simulink model "xEMU_SimulationModel3_rule1"  (R2017b)
settings: Solver=ode4  StartTime=0.0  StopTime=8192  FixedStep=0.01  RelTol=1e-3
undefined symbols (not defined in the file): a1, a2, a3, a4, ACO, BAT, Battery, DCT, DRT, EMS, ENV, Fahrzyklus_VS_modell, height_BAT, leistung, lib_bat, Maximum, Maximum_position, Num_cells, P_FC_max_long, P_FC_min_long, P_FC_step_max, Pbat_charge_max, Pbat_discharge_max, Pfc_max, Pfc_min, SOC_tar, time_peaks, TRM, velocity_peaks
libraries: simulink x5
(part 3 of 15)

== system xEMU_SimulationModel3_rule1/Battery (BAT)_mittel_02/Cell/Thermal ==
  CellToFV : Subsystem
  ConductivityMatrix : MATLAB Function  TreatAsAtomicUnit=on
  Coolings : Subsystem
  FV Temperatures : Integrator  ExternalReset=rising  InitialCondition=[ MDL.battery.initialState.CellElement_1.temperature MDL.battery.initialState.CellElement_1.temperature MDL.battery.initialState.CellElement_1.temperature MDL.battery.initialState.CellElement_1.temperature MDL.battery.initialState.CellElement_1.temperature MDL.battery.initialState.CellElement_1.temperature MDL.battery.initialState.CellElement_1.temperature MDL.battery.initialState.CellElement_1.temperature MDL.battery.initialState.CellElement_1.temperature MDL.battery.initialState.CellElement_1.temperature MDL.battery.initialState.CellElement_1.temperature MDL.battery.initialState.CellElement_1.temperature MDL.battery.initialState.CellElement_1.temperature MDL.battery.initialState.CellElement_1.temperature MDL.battery.initialState.CellElement_1.temperature MDL.battery.initialState.CellElement_1.temperature MDL.battery.initialState.CellElement_1.temperature MDL.battery.initialState.CellElement_1.temperature MDL.battery.initialState.CellElement_1.temperature MDL.battery.initialState.CellElement_1.temperature MDL.battery.initialState.CellElement_1.temperature MDL.battery.initialState.CellElement_1.temperature MDL.battery.initialState.CellElement_1.temperature MDL.battery.initialState.CellElement_1.temperature MDL.battery.initialState.CellElement_1.temperature MDL.battery.initialState.CellElement_1.temperature MDL.battery.initialState.CellElement_1.temperature MDL.battery.initialState.CellElement_1.temperature MDL.battery.initialState.CellElement_1.temperature MDL.battery.initialState.CellElement_1.temperature MDL.battery.initialState.CellElement_1.temperature MDL.battery.initialState.CellElement_1.temperature MDL.battery.initialState.CellElement_1.temperature MDL.battery.initialState.CellElement_1.temperature MDL.battery.initialState.CellElement_1.temperature MDL.battery.initialState.CellElement_1.temperature MDL.battery.initialState.CellElement_1.temperature MDL.battery.initialState.CellElement_1.temperature MDL.battery.initialState.CellElement_1.temperature MDL.battery.initialState.CellElement_1.temperature MDL.battery.initialState.CellElement_1.temperature MDL.battery.initialState.CellElement_1.temperature MDL.battery.initialState.CellElement_1.temperature MDL.battery.initialState.CellElement_1.temperature MDL.battery.initialState.CellElement_1.temperature MDL.battery.initialState.CellElement_1.temperature MDL.battery.initialState.CellElement_1.temperature MDL.battery.initialState.CellElement_1.temperature MDL.battery.initialState.CellElement_1.temperature MDL.battery.initialState.CellElement_1.temperature MDL.battery.initialState.CellElement_1.temperature MDL.battery.initialState.CellElement_1.temperature MDL.battery.initialState.CellElement_1.temperature MDL.battery.initialState.CellElement_1.temperature MDL.battery.initialState.CellElement_1.temperature MDL.battery.initialState.CellElement_1.temperature MDL.battery.initialState.CellElement_1.temperature MDL.battery.initialState.CellElement_1.temperature MDL.battery.initialState.CellElement_1.temperature MDL.battery.initialState.CellElement_1.temperature MDL.battery.initialState.CellElement_1.temperature MDL.battery.initialState.CellElement_1.temperature MDL.battery.initialState.CellElement_1.temperature MDL.battery.initialState.CellElement_1.temperature MDL.battery.initialState.CellElement_1.temperature MDL.battery.initialState.CellElement_1.temperature MDL.battery.initialState.CellElement_1.temperature MDL.battery.initialState.CellElement_1.temperature MDL.battery.initialState.CellElement_1.temperature MDL.battery.initialState.CellElement_1.temperature MDL.battery.initialState.CellElement_1.temperature MDL.battery.initialState.CellElement_1.temperature MDL.battery.initialState.CellElement_1.temperature MDL.battery.initialState.CellElement_1.temperature MDL.battery.initialState.CellElement_1.temperature MDL.battery.initialState.CellElement_1.temperature MDL.battery.initialState.CellElement_1.temperature MDL.battery.initialState.CellElement_1.temperature MDL.battery.initialState.CellElement_1.temperature MDL.battery.initialState.CellElement_1.temperature MDL.battery.initialState.CellElement_1.temperature MDL.battery.initialState.CellElement_1.temperature MDL.battery.initialState.CellElement_1.temperature MDL.battery.initialState.CellElement_1.temperature MDL.battery.initialState.CellElement_1.temperature MDL.battery.initialState.CellElement_1.temperature MDL.battery.initialState.CellElement_1.temperature MDL.battery.initialState.CellElement_1.temperature MDL.battery.initialState.CellElement_1.temperature MDL.battery.initialState.CellElement_1.temperature MDL.battery.initialState.CellElement_1.temperature MDL.battery.initialState.CellElement_1.temperature MDL.battery.initialState.CellElement_1.temperature MDL.battery.initialState.CellElement_1.temperature MDL.battery.initialState.CellElement_1.temperature MDL.battery.initialState.CellElement_1.temperature MDL.battery.initialState.CellElement_1.temperature MDL.battery.initialState.CellElement_1.temperature MDL.battery.initialState.CellElement_1.temperature MDL.battery.initialState.CellElement_1.temperature MDL.battery.initialState.CellElement_1.temperature MDL.battery.initialState.CellElement_1.temperature MDL.battery.initialState.CellElement_1.temperature MDL.battery.initialState.CellElement_1.temperature MDL.battery.initialState.CellElement_1.temperature MDL.battery.initialState.CellElement_1.temperature MDL.battery.initialState.CellElement_1.temperature MDL.battery.initialState.CellElement_1.temperature MDL.battery.initialState.CellElement_1.temperature MDL.battery.initialState.CellElement_1.temperature MDL.battery.initialState.CellElement_1.temperature MDL.battery.initialState.CellElement_1.temperature MDL.battery.initialState.CellElement_1.temperature MDL.battery.initialState.CellElement_1.temperature MDL.battery.initialState.CellElement_1.temperature MDL.battery.initialState.CellElement_1.temperature MDL.battery.initialState.CellElement_1.temperature MDL.battery.initialState.CellElement_1.temperature MDL.battery.initialState.CellElement_1.temperature MDL.battery.initialState.CellElement_1.temperature MDL.battery.initialState.CellElement_1.temperature MDL.battery.initialState.CellElement_1.temperature MDL.battery.initialState.CellElement_1.temperature MDL.battery.initialState.CellElement_1.temperature MDL.battery.initialState.CellElement_1.temperature MDL.battery.initialState.CellElement_1.temperature MDL.battery.initialState.CellElement_1.temperature MDL.battery.initialState.CellElement_1.temperature MDL.battery.initialState.CellElement_1.temperature MDL.battery.initialState.CellElement_1.temperature MDL.battery.initialState.CellElement_1.temperature MDL.battery.initialState.CellElement_1.temperature MDL.battery.initialState.CellElement_1.temperature MDL.battery.initialState.CellElement_1.temperature MDL.battery.initialState.CellElement_1.temperature MDL.battery.initialState.CellElement_1.temperature MDL.battery.initialState.CellElement_1.temperature MDL.battery.initialState.CellElement_1.temperature MDL.battery.initialState.CellElement_1.temperature MDL.battery.initialState.CellElement_1.temperature MDL.battery.initialState.CellElement_1.temperature MDL.battery.initialState.CellElement_1.temperature MDL.battery.initialState.CellElement_1.temperature MDL.battery.initialState.CellElement_1.temperature MDL.battery.initialState.CellElement_1.temperature MDL.battery.initialState.CellElement_1.temperature MDL.battery.initialState.CellElement_1.temperature MDL.battery.initialState.CellElement_1.temperature MDL.battery.initialState.CellElement_1.temperature MDL.battery.initialState.CellElement_1.temperature MDL.battery.initialState.CellElement_1.temperature MDL.battery.initialState.CellElement_1.temperature MDL.battery.initialState.CellElement_1.temperature MDL.battery.initialState.CellElement_1.temperature MDL.battery.initialState.CellElement_1.temperature MDL.battery.initialState.CellElement_1.temperature MDL.battery.initialState.CellElement_1.temperature MDL.battery.initialState.CellElement_1.temperature MDL.battery.initialState.CellElement_1.temperature MDL.battery.initialState.CellElement_1.temperature MDL.battery.initialState.CellElement_1.temperature MDL.battery.initialState.CellElement_1.temperature MDL.battery.initialState.CellElement_1.temperature MDL.battery.initialState.CellElement_1.temperature MDL.battery.initialState.CellElement_1.temperature MDL.battery.initialState.CellElement_1.temperature MDL.battery.initialState.CellElement_1.temperature MDL.battery.initialState.CellElement_1.temperature MDL.battery.initialState.CellElement_1.temperature MDL.battery.initialState.CellElement_1.temperature MDL.battery.initialState.CellElement_1.temperature MDL.battery.initialState.CellElement_1.temperature MDL.battery.initialState.CellElement_1.temperature MDL.battery.initialState.CellElement_1.temperature MDL.battery.initialState.CellElement_1.temperature MDL.battery.initialState.CellElement_1.temperature MDL.battery.initialState.CellElement_1.temperature MDL.battery.initialState.CellElement_1.temperature MDL.battery.initialState.CellElement_1.temperature MDL.battery.initialState.CellElement_1.temperature MDL.battery.initialState.CellElement_1.temperature MDL.battery.initialState.CellElement_1.temperature MDL.battery.initialState.CellElement_1.temperature MDL.battery.initialState.CellElement_1.temperature MDL.battery.initialState.CellElement_1.temperature MDL.battery.initialState.CellElement_1.temperature MDL.battery.initialState.CellElement_1.temperature MDL.battery.initialState.CellElement_1.temperature MDL.battery.initialState.CellElement_1.temperature MDL.battery.initialState.CellElement_1.temperature MDL.battery.initialState.CellElement_1.temperature MDL.battery.initialState.CellElement_1.temperature MDL.battery.initialState.CellElement_1.temperature MDL.battery.initialState.CellElement_1.temperature MDL.battery.initialState.CellElement_1.temperature MDL.battery.initialState.CellElement_1.temperature MDL.battery.initialState.CellElement_1.temperature MDL.battery.initialState.CellElement_1.temperature MDL.battery.initialState.CellElement_1.temperature MDL.battery.initialState.CellElement_1.temperature MDL.battery.initialState.CellElement_1.temperature MDL.battery.initialState.CellElement_1.temperature MDL.battery.initialState.CellElement_1.temperature MDL.battery.initialState.CellElement_1.temperature MDL.battery.initialState.CellElement_1.temperature MDL.battery.initialState.CellElement_1.temperature MDL.battery.initialState.CellElement_1.temperature MDL.battery.initialState.CellElement_1.temperature MDL.battery.initialState.CellElement_1.temperature MDL.battery.initialState.CellElement_1.temperature MDL.battery.initialState.CellElement_1.temperature MDL.battery.initialState.CellElement_1.temperature MDL.battery.initialState.CellElement_1.temperature MDL.battery.initialState.CellElement_1.temperature MDL.battery.initialState.CellElement_1.temperature MDL.battery.initialState.CellElement_1.temperature MDL.battery.initialState.CellElement_1.temperature MDL.battery.initialState.CellElement_1.temperature MDL.battery.initialState.CellElement_1.temperature MDL.battery.initialState.CellElement_1.temperature MDL.battery.initialState.CellElement_1.temperature MDL.battery.initialState.CellElement_1.temperature MDL.battery.initialState.CellElement_1.temperature MDL.battery.initialState.CellElement_1.temperature MDL.battery.initialState.CellElement_1.temperature MDL.battery.initialState.CellElement_1.temperature MDL.battery.initialState.CellElement_1.temperature MDL.battery.initialState.CellElement_1.temperature MDL.battery.initialState.CellElement_1.temperature MDL.battery.initialState.CellElement_1.temperature MDL.battery.initialState.CellElement_1.temperature MDL.battery.initialState.CellElement_1.temperature MDL.battery.initialState.CellElement_1.temperature MDL.battery.initialState.CellElement_1.temperature MDL.battery.initialState.CellElement_1.temperature MDL.battery.initialState.CellElement_1.temperature MDL.battery.initialState.CellElement_1.temperature MDL.battery.initialState.CellElement_1.temperature MDL.battery.initialState.CellElement_1.temperature MDL.battery.initialState.CellElement_1.temperature MDL.battery.initialState.CellElement_1.temperature MDL.battery.initialState.CellElement_1.temperature MDL.battery.initialState.CellElement_1.temperature MDL.battery.initialState.CellElement_1.temperature MDL.battery.initialState.CellElement_1.temperature MDL.battery.initialState.CellElement_1.temperature MDL.battery.initialState.CellElement_1.temperature MDL.battery.initialState.CellElement_1.temperature MDL.battery.initialState.CellElement_1.temperature MDL.battery.initialState.CellElement_1.temperature MDL.battery.initialState.CellElement_1.temperature MDL.battery.initialState.CellElement_1.temperature MDL.battery.initialState.CellElement_1.temperature MDL.battery.initialState.CellElement_1.temperature MDL.battery.initialState.CellElement_1.temperature MDL.battery.initialState.CellElement_1.temperature MDL.battery.initialState.CellElement_1.temperature MDL.battery.initialState.CellElement_1.temperature MDL.battery.initialState.CellElement_1.temperature MDL.battery.initialState.CellElement_1.temperature MDL.battery.initialState.CellElement_1.temperature MDL.battery.initialState.CellElement_1.temperature MDL.battery.initialState.CellElement_1.temperature MDL.battery.initialState.CellElement_1.temperature MDL.battery.initialState.CellElement_1.temperature MDL.battery.initialState.CellElement_1.temperature MDL.battery.initialState.CellElement_1.temperature MDL.battery.initialState.CellElement_1.temperature MDL.battery.initialState.CellElement_1.temperature MDL.battery.initialState.CellElement_1.temperature MDL.battery.initialState.CellElement_1.temperature MDL.battery.initialState.CellElement_1.temperature MDL.battery.initialState.CellElement_1.temperature MDL.battery.initialState.CellElement_1.temperature MDL.battery.initialState.CellElement_1.temperature MDL.battery.initialState.CellElement_1.temperature MDL.battery.initialState.CellElement_1.temperature MDL.battery.initialState.CellElement_1.temperature MDL.battery.initialState.CellElement_1.temperature MDL.battery.initialState.CellElement_1.temperature MDL.battery.initialState.CellElement_1.temperature MDL.battery.initialState.CellElement_1.temperature MDL.battery.initialState.CellElement_1.temperature MDL.battery.initialState.CellElement_1.temperature MDL.battery.initialState.CellElement_1.temperature MDL.battery.initialState.CellElement_1.temperature MDL.battery.initialState.CellElement_1.temperature MDL.battery.initialState.CellElement_1.temperature MDL.battery.initialState.CellElement_1.temperature MDL.battery.initialState.CellElement_1.temperature MDL.battery.initialState.CellElement_1.temperature MDL.battery.initialState.CellElement_1.temperature MDL.battery.initialState.CellElement_1.temperature MDL.battery.initialState.CellElement_1.temperature MDL.battery.initialState.CellElement_1.temperature MDL.battery.initialState.CellElement_1.temperature MDL.battery.initialState.CellElement_1.temperature MDL.battery.initialState.CellElement_1.temperature MDL.battery.initialState.CellElement_1.temperature MDL.battery.initialState.CellElement_1.temperature ]
  FVToCell : Subsystem
  Reciprocals of Thermal Capacities : Gain  Gain=[0.582768314846317;0.582768314846317;0.582768314846317;0.582768314846317;0.582768314846317;0.582768314846317;0.582768314846317;0.582768314846317;0.582768314846317;0.582768314846317;0.582768314846317;0.582768314846317;0.582768314846317;0.582768314846317;0.582768314846317;0.582768314846317;0.582768314846317;0.582768314846317;0.582768314846317;0.582768314846317;0.582768314846317;0.582768314846317;0.582768314846317;0.582768314846317;0.582768314846317;0.582768314846317;0.582768314846317;0.582768314846317;0.582768314846317;0.582768314846317;0.582768314846317;0.582768314846317;0.582768314846317;0.582768314846317;0.582768314846317;0.582768314846317;0.582768314846317;0.582768314846317;0.582768314846317;0.582768314846317;0.582768314846317;0.582768314846317;0.582768314846317;0.582768314846317;0.582768314846317;0.582768314846317;0.582768314846317;0.582768314846317;0.582768314846317;0.582768314846317;0.582768314846317;0.582768314846317;0.582768314846317;0.582768314846317;0.582768314846317;0.582768314846317;0.582768314846317;0.582768314846317;0.582768314846317;0.582768314846317;0.582768314846317;0.582768314846317;0.582768314846317;0.582768314846317;0.582768314846317;0.582768314846317;0.582768314846317;0.582768314846317;0.582768314846317;0.582768314846317;0.582768314846317;0.582768314846317;0.582768314846317;0.582768314846317;0.582768314846317;0.582768314846317;0.582768314846317;0.582768314846317;0.582768314846317;0.582768314846317;0.582768314846317;0.582768314846317;0.582768314846317;0.582768314846317;0.582768314846317;0.582768314846317;0.582768314846317;0.582768314846317;0.582768314846317;0.582768314846317;0.582768314846317;0.582768314846317;0.582768314846317;0.582768314846317;0.582768314846317;0.582768314846317;0.582768314846317;0.582768314846317;0.582768314846317;0.582768314846317;0.582768314846317;0.582768314846317;0.582768314846317;0.582768314846317;0.582768314846317;0.582768314846317;0.582768314846317;0.582768314846317;0.582768314846317;0.582768314846317;0.582768314846317;0.582768314846317;0.582768314846317;0.582768314846317;0.582768314846317;0.582768314846317;0.582768314846317;0.582768314846317;0.582768314846317;0.582768314846317;0.582768314846317;0.582768314846317;0.582768314846317;0.582768314846317;0.582768314846317;0.582768314846317;0.582768314846317;0.582768314846317;0.582768314846317;0.582768314846317;0.582768314846317;0.582768314846317;0.582768314846317;0.582768314846317;0.582768314846317;0.582768314846317;0.582768314846317;0.582768314846317;0.582768314846317;0.582768314846317;0.582768314846317;0.582768314846317;0.582768314846317;0.582768314846317;0.582768314846317;0.582768314846317;0.582768314846317;0.582768314846317;0.582768314846317;0.582768314846317;0.582768314846317;0.582768314846317;0.582768314846317;0.582768314846317;0.582768314846317;0.582768314846317;0.582768314846317;0.582768314846317;0.582768314846317;0.582768314846317;0.582768314846317;0.582768314846317;0.582768314846317;0.582768314846317;0.582768314846317;0.582768314846317;0.582768314846317;0.582768314846317;0.582768314846317;0.582768314846317;0.582768314846317;0.582768314846317;0.582768314846317;0.582768314846317;0.582768314846317;0.582768314846317;0.582768314846317;0.582768314846317;0.582768314846317;0.582768314846317;0.582768314846317;0.582768314846317;0.582768314846317;0.582768314846317;0.582768314846317;0.582768314846317;0.582768314846317;0.582768314846317;0.582768314846317;0.582768314846317;0.582768314846317;0.582768314846317;0.582768314846317;0.582768314846317;0.582768314846317;0.582768314846317;0.582768314846317;0.582768314846317;0.582768314846317;0.582768314846317;0.582768314846317;0.582768314846317;0.582768314846317;0.582768314846317;0.582768314846317;0.582768314846317;0.582768314846317;0.582768314846317;0.582768314846317;0.582768314846317;0.582768314846317;0.582768314846317;0.582768314846317;0.582768314846317;0.582768314846317;0.582768314846317;0.582768314846317;0.582768314846317;0.582768314846317;0.582768314846317;0.582768314846317;0.582768314846317 ...(+1404 chars)]
  Sum : Sum  Inputs=|+-+
  wires:
  [Reset] -> FV Temperatures/2
  ConductivityMatrix/1(y) -> Sum/3
  CellToFV/1(P_FV) -> Sum/1
  Coolings/1(P_FV) -> Sum/2
  FV Temperatures/1 -> Coolings/1(T_FV), ConductivityMatrix/1(u), FVToCell/1(T_FV)
  Reciprocals of Thermal Capacities/1 -> FV Temperatures/1
  Sum/1 -> Reciprocals of Thermal Capacities/1

== system xEMU_SimulationModel3_rule1/Battery (BAT)_mittel_02/Cell/TotalValues ==
  Component0 : Subsystem
  Component1 : Subsystem
  Component2 : Subsystem
  Current : Outport
  Voltage : Outport  Port=2
  Power : Outport  Port=3
  wires:
  Component0/3(Value) -> Current/1
  Component1/3(Value) -> Voltage/1
  Component2/3(Value) -> Power/1

== system xEMU_SimulationModel3_rule1/DCDC Traction (DCT)/DCDC_elektrisch_Modellierung/Efficiency measurment ==
  In1 : Inport
  In2 : Inport  Port=2
  Abs : Abs
  Abs1 : Abs
  Clock : Clock
  Constant : Constant
  Constant1 : Constant  Value=0
  Divide : Product  Inputs=*/
  Divide1 : Product  Inputs=*/
  Divide2 : Product  Inputs=*/
  Integrator2 : Integrator
  Relational Operator : RelationalOperator  Operator=<=  OutDataTypeStr=boolean  RndMeth=Simplest
  Relational Operator1 : RelationalOperator  Operator===  OutDataTypeStr=boolean  RndMeth=Simplest
  Scope : Scope  NumInputPorts=4
  Switch : Switch  Criteria=u2 > Threshold
  Switch1 : Switch  Criteria=u2 > Threshold
  Efficiency : Outport
  wires:
  Abs/1 -> Divide/2, Divide1/1, Relational Operator/1
  In2/1 -> Scope/2, Abs1/1
  Abs1/1 -> Divide1/2, Relational Operator/2, Divide/1
  Switch1/1 -> Integrator2/1, Scope/4
  Relational Operator1/1 -> Switch1/2
  In1/1 -> Scope/1, Abs/1
  Divide1/1 -> Switch/1
  Divide/1 -> Switch/3
  Constant1/1 -> Relational Operator1/1
  Relational Operator/1 -> Switch/2
  Switch/1 -> Switch1/3, Relational Operator1/2, Scope/3
  Constant/1 -> Switch1/1
  Integrator2/1 -> Divide2/1
  Clock/1 -> Divide2/2
  Divide2/1 -> Efficiency/1

== system xEMU_SimulationModel3_rule1/DCDC Traction (DCT)/DCDC_elektrisch_Modellierung/Efficiency measurment1 ==
  In1 : Inport
  In2 : Inport  Port=2
  Abs : Abs
  Abs1 : Abs
  Divide3 : Product  Inputs=*/
  Integrator1 : Integrator
  Integrator3 : Integrator
  Sum : Sum  Inputs=|++
  Switch1 : Switch
  Switch2 : Switch
  Efficiency : Outport
  wires:
  In2/1 -> Sum/2
  Sum/1 -> Abs/1
  Abs1/1 -> Switch1/3, Switch2/1
  In1/1 -> Abs1/1, Switch2/2, Switch1/2, Sum/1
  Switch1/1 -> Integrator1/1
  Abs/1 -> Switch2/3, Switch1/1
  Switch2/1 -> Integrator3/1
  Integrator3/1 -> Divide3/1
  Integrator1/1 -> Divide3/2
  Divide3/1 -> Efficiency/1

== system xEMU_SimulationModel3_rule1/Drive Train (DRT)/Converter and traction motor/Converter_DRT ==
  "I_traction_motor " : Inport
  V_dcLinkStorage_V : Inport  Port=2
  V_Drive_V : Inport  Port=3
  Cos_Phi_Phaseshift : Inport  Port=4
  RPM : Inport  Port=5
  Clock : Clock
  Display : Display
  Divide2 : Product  Inputs=*/
  Gain : Gain  Gain=1/1000
  Gain3 : Gain  Gain=1/sqrt(3)
  Integrator2 : Integrator
  Sum : Sum  Inputs=|++
  n-D Lookup Diode : Lookup_n-D  NumberOfTableDimensions=4  BreakpointsForDimension1=DRT.converter.loss_diode.D1_U_Load  BreakpointsForDimension2=DRT.converter.loss_diode.D2_I_Load  BreakpointsForDimension3=DRT.converter.loss_diode.D3_rpm  BreakpointsForDimension4=DRT.converter.loss_diode.D4_P_Factor  Table=DRT.converter.loss_diode.loss  InternalRulePriority=Speed  RndMeth=Simplest  InputSameDT=on
  n-D Lookup Efficiency : Lookup_n-D  NumberOfTableDimensions=4  BreakpointsForDimension1=DRT.converter.efficiency.D1_U_Load  BreakpointsForDimension2=DRT.converter.efficiency.D2_I_Load  BreakpointsForDimension3=DRT.converter.efficiency.D3_rpm  BreakpointsForDimension4=DRT.converter.efficiency.D4_P_Factor  Table=DRT.converter.efficiency.efficiency  InternalRulePriority=Speed  RndMeth=Simplest  InputSameDT=on
  n-D Lookup IGBT : Lookup_n-D  NumberOfTableDimensions=4  BreakpointsForDimension1=DRT.converter.loss_igbt.D1_U_Load  BreakpointsForDimension2=DRT.converter.loss_igbt.D2_I_Load  BreakpointsForDimension3=DRT.converter.loss_igbt.D3_rpm  BreakpointsForDimension4=DRT.converter.loss_igbt.D4_P_Factor  Table=DRT.converter.loss_igbt.loss  InternalRulePriority=Speed  RndMeth=Simplest  InputSameDT=on
  P_dcLinkTractionLoss_kW : Outport
  Efficiency_out : Outport  Port=2
  wires:
  Gain/1 -> P_dcLinkTractionLoss_kW/1
  "I_traction_motor "/1 -> n-D Lookup IGBT/2, n-D Lookup Efficiency/2, n-D Lookup Diode/2  "I_tractionmotor"
  Sum/1 -> Gain/1
  n-D Lookup IGBT/1 -> Sum/1
  n-D Lookup Diode/1 -> Sum/2
  V_Drive_V/1 -> Gain3/1
  Gain3/1 -> n-D Lookup Efficiency/1, n-D Lookup Diode/1, n-D Lookup IGBT/1
  Cos_Phi_Phaseshift/1 -> n-D Lookup Efficiency/4, n-D Lookup IGBT/4, n-D Lookup Diode/4
  RPM/1 -> n-D Lookup Efficiency/3, n-D Lookup Diode/3, n-D Lookup IGBT/3
  V_dcLinkStorage_V/1 -> Display/1
  Clock/1 -> Divide2/2
  Integrator2/1 -> Divide2/1
  n-D Lookup Efficiency/1 -> Integrator2/1
  Divide2/1 -> Efficiency_out/1

== system xEMU_SimulationModel3_rule1/Drive Train (DRT)/Converter and traction motor/Efficiency measurment1 ==
  In1 : Inport
  In2 : Inport  Port=2
  Abs : Abs
  Abs1 : Abs
  Divide3 : Product  Inputs=*/
  Integrator1 : Integrator
  Integrator3 : Integrator
  Sum : Sum  Inputs=|++
  Switch1 : Switch
  Switch2 : Switch
  Efficiency : Outport
  wires:
  In2/1 -> Sum/2
  Sum/1 -> Abs/1
  Abs1/1 -> Switch1/3, Switch2/1
  In1/1 -> Abs1/1, Switch2/2, Switch1/2, Sum/1
  Switch1/1 -> Integrator1/1
  Abs/1 -> Switch2/3, Switch1/1
  Switch2/1 -> Integrator3/1
  Integrator3/1 -> Divide3/1
  Integrator1/1 -> Divide3/2
  Divide3/1 -> Efficiency/1

== system xEMU_SimulationModel3_rule1/Drive Train (DRT)/Converter and traction motor/traction_motor_kennfeldbasiert ==
  M_soll : Inport
  n : Inport  Port=2
  2-D I_strang_kombi_motor_generator : Lookup_n-D  BreakpointsForDimension1=torquevector  BreakpointsForDimension2=speedvector  Table=I_strang  InternalRulePriority=Speed  RndMeth=Simplest  InputSameDT=on
  2-D Pv_motor : Lookup_n-D  BreakpointsForDimension1=torquevector  BreakpointsForDimension2=speedvector  Table=Pv_motor  ExtrapMethod=Clip  UseLastTableValue=on  InternalRulePriority=Speed  RndMeth=Simplest  InputSameDT=on
  2-D U_LL_kombi_motor_generator : Lookup_n-D  BreakpointsForDimension1=torquevector  BreakpointsForDimension2=speedvector  Table=U_LL  InternalRulePriority=Speed  RndMeth=Simplest  InputSameDT=on
  2-D cosphi2_kombi_motor_generator : Lookup_n-D  BreakpointsForDimension1=torquevector2  BreakpointsForDimension2=speedvector2  Table=cosphi2  InternalRulePriority=Speed  RndMeth=Simplest  InputSameDT=on
  Add : Sum
  Gain1 : Gain  Gain=sqrt(2)
  Gain10 : Gain  Gain=1/1000
  Gain2 : Gain  Gain=1/1000
  Gain3 : Gain  Gain=sqrt(3)
  Gain4 : Gain  Gain=0.99
  Gain5 : Gain  Gain=0.99
  Gain6 : Gain  Gain=sqrt(2)
  Gain8 : Gain  Gain=2*pi/60
  MATLAB Function1 : MATLAB Function  TreatAsAtomicUnit=on
  M_obergenze : Lookup_n-D  NumberOfTableDimensions=1  BreakpointsForDimension1=speedvector  Table=torque_obergrenze  InternalRulePriority=Speed  RndMeth=Simplest  InputSameDT=on
  M_untergenze : Lookup_n-D  NumberOfTableDimensions=1  BreakpointsForDimension1=speedvector  Table=torque_untergrenze  InternalRulePriority=Speed  RndMeth=Simplest  InputSameDT=on
  Product4 : Product
  Subsystem : Subsystem
  Subsystem1 : Subsystem
  Subsystem2 : Subsystem
  Subsystem3 : Subsystem
  "wegen extrapolation ist manche werte der lookuptable fehlerbehaft " : Saturate  UpperLimit=1  LowerLimit=-1
  P_el : Outport
  M_ist : Outport  Port=2
  U_1 : Outport  Port=3
  I_1 : Outport  Port=4
  cos_phi : Outport  Port=5
  Pv_motor : Outport  Port=6
  tag scope: P_motor_mechanic=global
  wires:
  Gain10/1 -> Add/1, [P_motor_mechanic]
  Gain8/1 -> Product4/2
  Product4/1 -> Gain10/1
  2-D U_LL_kombi_motor_generator/1 -> Subsystem2/2("lookuptable_coshpi ")
  Gain6/1 -> U_1/1  "u_ll_scheitel"
  2-D I_strang_kombi_motor_generator/1 -> Subsystem3/2("lookuptable_coshpi ")
  Gain1/1 -> I_1/1  "I_leiter_scheitel"
  Gain2/1 -> Add/2, Pv_motor/1
  Add/1 -> P_el/1
  MATLAB Function1/1(M_ist) -> Product4/1, Subsystem/1(M), 2-D Pv_motor/1, Subsystem1/1(M), 2-D cosphi2_kombi_motor_generator/1, Subsystem3/1(M), 2-D I_strang_kombi_motor_generator/1, Subsystem2/1(M), 2-D U_LL_kombi_motor_generator/1, M_ist/1
  Gain3/1 -> Gain6/1
  M_obergenze/1 -> Gain4/1
  M_untergenze/1 -> Gain5/1
  Gain4/1 -> MATLAB Function1/3(M_max)
  Gain5/1 -> MATLAB Function1/2(M_min)
  "wegen extrapolation ist manche werte der lookuptable fehlerbehaft "/1 -> cos_phi/1
  M_soll/1 -> MATLAB Function1/1(M_soll)
  n/1 -> Subsystem1/3("n "), 2-D cosphi2_kombi_motor_generator/2, Subsystem3/3("n "), 2-D I_strang_kombi_motor_generator/2, Subsystem2/3("n "), 2-D U_LL_kombi_motor_generator/2, Subsystem/3("n "), 2-D Pv_motor/2, Gain8/1, M_obergenze/1, M_untergenze/1
  Subsystem/1(Pv_motor) -> Gain2/1
  2-D cosphi2_kombi_motor_generator/1 -> Subsystem1/2("lookuptable_coshpi ")
  2-D Pv_motor/1 -> Subsystem/2("lookuptable_Pv ")
  Subsystem3/1(I_strang_motor) -> Gain1/1
  Subsystem2/1(U_LL_motor) -> Gain3/1
  Subsystem1/1(coshpi_motor) -> "wegen extrapolation ist manche werte der lookuptable fehlerbehaft "/1

== system xEMU_SimulationModel3_rule1/Drive Train (DRT)/Slipmodel and Traction /Tire Resistance  ==
  numberdrivesavailable : Inport
  total mass_kg : Inport  Port=2
  f_traction_tire : Inport  Port=3
  Divide1 : Product  Inputs=/*
  Gain4 : Gain  Gain=R_wheel_drt_m
  Gain5 : Gain  Gain=g_drt/2
  resistance of tire : Outport
  Fz_tire : Outport  Port=2
  wires:
  Divide1/1 -> Gain5/1
  total mass_kg/1 -> Divide1/2
  numberdrivesavailable/1 -> Divide1/1
  Gain4/1 -> resistance of tire/1
  Gain5/1 -> Fz_tire/1
  f_traction_tire/1 -> Gain4/1

== system xEMU_SimulationModel3_rule1/Drive Train (DRT)/Slipmodel and Traction /Variant Subsystem1 ==
  note: 1) Add Subsystem or Model blocks as valid variant choices.
      | 2) You cannot connect blocks at this level. At simulation, connectivity is automatically
      | determined, based on the active variant and port name matching.
  T_EMAdemandper_axis_Nm : Inport
  v_train_m/s : Inport  Port=2
  adhesionCoefficient_abs : Inport  Port=3
  Resistance of tire : Inport  Port=4
  Fz_tire : Inport  Port=5
  Mit_Schlupf_nach_Kalker : Subsystem  VariantControl=Variant
  Mit_Schlupf_nach_Yoshiki : Subsystem  VariantControl=Variant1
  Ohne_Schlupf : Subsystem  VariantControl=Variant2
  F_traction_peraxis_N : Outport
  WheelSpeed_rad/s : Outport  Port=2
  f_traction_tire : Outport  Port=3

== system xEMU_SimulationModel3_rule1/Energy Manager (EMA)/Kern von EMS/Leistungsflussverteilug  ==
  note: Mode Bestimmung
  P_load : Inport
  "P_load_aver " : Inport  Port=2
  SoC : Inport  Port=3
  MATLAB Function1 : MATLAB Function  TreatAsAtomicUnit=on
  Relay2 : Relay  OnSwitchValue=a2  OffSwitchValue=a1  OnOutputValue=2  OffOutputValue=1
  Relay3 : Relay  OnSwitchValue=a4  OffSwitchValue=a3  OnOutputValue=3  OffOutputValue=2
  Scope : Scope
  Switch2 : Switch  Threshold=2
  P_FCdemand_kW : Outport
  wires:
  Relay2/1 -> Switch2/3, Switch2/2
  Relay3/1 -> Switch2/1
  Switch2/1 -> Scope/1, MATLAB Function1/2(Mode)
  P_load/1 -> MATLAB Function1/1(P_load)
  SoC/1 -> Relay2/1, MATLAB Function1/3(SOC), Relay3/1
  "P_load_aver "/1 -> P_FCdemand_kW/1

== system xEMU_SimulationModel3_rule1/Energy Manager (EMA)/Kern von EMS/P_load_aver ==
  V_SOLL : Inport
  SOC : Inport  Port=2
  Constant : Constant
  Constant1 : Constant  Value=leistung
  Constant2 : Constant  Value=SOC_tar
  Constant3 : Constant  Value=Maximum_position
  Constant4 : Constant  Value=Maximum
  Constant5 : Constant  Value=time_peaks
  Constant6 : Constant  Value=height_BAT
  Constant7 : Constant  Value=velocity_peaks
  Delay1 : Delay  DelayLength=1  InitialCondition=0
  Delay2 : Delay  DelayLength=1  InitialCondition=0
  Integrator : Integrator
  Integrator1 : Integrator
  MATLAB Function3 : MATLAB Function  TreatAsAtomicUnit=on
  P_load_aver : MATLAB Function  TreatAsAtomicUnit=on
  Subsystem : Subsystem
  P_load_mean : Outport
  wires:
  Integrator1/1 -> MATLAB Function3/5(t), P_load_aver/10(t)
  V_SOLL/1 -> P_load_aver/7(v), Delay1/1
  Delay1/1 -> P_load_aver/8(v_before)
  Delay2/1 -> P_load_aver/11(P_Demand_aver_before)
  Integrator/1 -> P_load_aver/9(P_Demand_total)
  Constant2/1 -> MATLAB Function3/1(SOC_tar)
  [distance] -> MATLAB Function3/4(distance)
  P_load_aver/1(P_Demand_aver_pred) -> P_load_mean/1, Delay2/1
  Constant/1 -> Integrator1/1
  [F_EMAdemand_N] -> Subsystem/1(F_EMAdemand_N)
  [gradient] -> Subsystem/2(Gradient_force)
  [n_motor_rpm] -> Subsystem/3(n_motor_rpm)
  Subsystem/1(korrigierte_Pload) -> Integrator/1
  SOC/1 -> MATLAB Function3/3(SOC_current)
  Constant1/1 -> P_load_aver/6(leistung)
  [distance] -> P_load_aver/5(distance)
  Constant3/1 -> P_load_aver/4(peak_positions)
  Constant5/1 -> P_load_aver/3(time)
  Constant4/1 -> P_load_aver/2(height)
  Constant6/1 -> P_load_aver/1(height_bat)
  Constant7/1 -> P_load_aver/12(v_peak)

== system xEMU_SimulationModel3_rule1/Energy Manager (EMA)/Kern von EMS/Subsystem ==
  P_load_wunsch_kw : Inport
  P_fc_kann : Inport  Port=2
  SOC : Inport  Port=3
  <V_bat_V> : Inport  Port=4
  Ausschaltung der Batterie : MATLAB Function  TreatAsAtomicUnit=on
  Divide1 : Product  Inputs=*/
  I_bat_max_limits1 : Saturate  UpperLimit=EMS.Bat.I_discharge_max/1000  LowerLimit=-EMS.Bat.I_charge_max/1000
  Product1 : Product
  Rate Limiter : RateLimiter  RisingSlewLimit=EMS.Bat.I_change_rate  FallingSlewLimit=-EMS.Bat.I_change_rate  SampleTimeMode=inherited
  Scope : Scope
  Subtract : Sum  Inputs=-+
  P_bat_kann : Outport
  wires:
  Subtract/1 -> Ausschaltung der Batterie/2(Pbat)
  Ausschaltung der Batterie/1(P_bat) -> Divide1/1
  <V_bat_V>/1 -> Product1/2, Divide1/2
  P_fc_kann/1 -> Subtract/1
  P_load_wunsch_kw/1 -> Subtract/2
  SOC/1 -> Ausschaltung der Batterie/1(SoC)
  Product1/1 -> P_bat_kann/1  "P_bat_kann"
  Divide1/1 -> I_bat_max_limits1/1
  I_bat_max_limits1/1 -> Rate Limiter/1, Scope/1
  Rate Limiter/1 -> Product1/1

== system xEMU_SimulationModel3_rule1/Train Dynamics (TRM)/Variant Subsystem/v_s_model ==
  n_passengers_abs : Inport
  adhesionCoefficient_abs : Inport  Port=2
  F_traction_N : Inport  Port=3
  Bus Creator : BusCreator  Inputs=3
  Driver1 : Subsystem
  Driving Resistances : Subsystem
  Train Longitudinal Dynamics : Subsystem
  TRM_BUS : Outport
  F_tractionDemand_N : Outport  Port=2
  v_train_m/s : Outport  Port=3
  adhesionCoefficient : Outport  Port=4
  total_mass_kg : Outport  Port=5
  v_soll : Outport  Port=6
  wires:
  Driver1/1(F_tractionDemand_N) -> F_tractionDemand_N/1, Bus Creator/1  "F_tractionDemand_N"
  Driving Resistances/1(Fahrwiderstand_N) -> Train Longitudinal Dynamics/3(Fahrwiderstand_N), Bus Creator/3  "Fahrwiderstand"
  adhesionCoefficient_abs/1 -> adhesionCoefficient/1
  Train Longitudinal Dynamics/2(v_train_m/s) -> Driver1/2(v_train), v_train_m/s/1, Bus Creator/2, Driving Resistances/1(v_train)  "v_train_m/s"
  n_passengers_abs/1 -> Train Longitudinal Dynamics/1(n_passengers_abs)
  F_traction_N/1 -> Train Longitudinal Dynamics/2(F_traction_N)
  Bus Creator/1 -> TRM_BUS/1
  Train Longitudinal Dynamics/3(total_mass_kg) -> Driving Resistances/2(total mass), total_mass_kg/1
  Train Longitudinal Dynamics/1(v_soll_m/s) -> v_soll/1, Driver1/1(v_drivingCycle_m/s)
  Train Longitudinal Dynamics/4(Steigung_soll) -> Driving Resistances/3(gradient)

== system xEMU_SimulationModel3_rule1/Train Dynamics (TRM)/Variant Subsystem/v_t_model ==
  v_drivingCycle_m/s : Inport
  h_drivingCycle_m : Inport  Port=2
  n_passengers_abs : Inport  Port=3
  adhesionCoefficient_abs : Inport  Port=4
  F_traction_N : Inport  Port=5
  Bus Creator : BusCreator  Inputs=3
  Driver1 : Subsystem
  Driving Resistances : Subsystem
  Train Longitudinal Dynamics : Subsystem
  TRM_BUS : Outport
  F_tractionDemand_N : Outport  Port=2
  v_train_m/s : Outport  Port=3
  adhesionCoefficient : Outport  Port=4
  total_mass_kg : Outport  Port=5
  v_soll : Outport  Port=6
  wires:
  n_passengers_abs/1 -> Train Longitudinal Dynamics/2(n_passengers_abs)
  adhesionCoefficient_abs/1 -> adhesionCoefficient/1
  Driver1/1(F_tractionDemand_N) -> F_tractionDemand_N/1, Bus Creator/3  "F_tractionDemand_N"
  Bus Creator/1 -> TRM_BUS/1
  Driving Resistances/1(air&gradient_resistance_N) -> Bus Creator/2, Train Longitudinal Dynamics/1(air&gradient_resistance_N)  "Fahrwiderstand"
  Train Longitudinal Dynamics/1(total_mass_kg) -> Driving Resistances/3(total mass), total_mass_kg/1
  F_traction_N/1 -> Train Longitudinal Dynamics/3(F_traction_N)
  Train Longitudinal Dynamics/2(v_train_m/s) -> v_train_m/s/1, Bus Creator/1, Driving Resistances/1(v_train), Driver1/2(v_train)  "v_train_m/s"
  v_drivingCycle_m/s/1 -> v_soll/1, Driver1/1(v_drivingCycle_m/s)
  h_drivingCycle_m/1 -> Driving Resistances/2(gradient)

== system xEMU_SimulationModel3_rule1/Battery (BAT)_komplex/Subsystem/CellCurrentMatrices/Component0 ==
  ColConst : Constant  Value=0
  RowConst : Constant  Value=0
  Row : Outport
  Col : Outport  Port=2
  Value : Outport  Port=3
  wires:
  ColConst/1 -> Col/1
  RowConst/1 -> Row/1
  [InputCurrent] -> Value/1

== system xEMU_SimulationModel3_rule1/Battery (BAT)_komplex/Subsystem/CellCurrentMatrices/Component1 ==
  ColConst : Constant  Value=0
  RowConst : Constant  Value=0
  Row : Outport
  Col : Outport  Port=2
  Value : Outport  Port=3
  wires:
  ColConst/1 -> Col/1
  RowConst/1 -> Row/1
  [InputCurrent] -> Value/1

== system xEMU_SimulationModel3_rule1/Battery (BAT)_komplex/Subsystem/CellVoltageMatrices/Component0 ==
  Add10_1 : Sum
  Add11_1 : Sum
  Add12_1 : Sum
  Add13_1 : Sum
  Add14_1 : Sum
  Add15_1 : Sum
  Add15_4 : Sum
  Add16_1 : Sum
  Add16_3 : Sum
  Add16_4 : Sum
  Add17_1 : Sum
  Add17_3 : Sum
  Add18_1 : Sum
  Add18_3 : Sum
  Add19_1 : Sum
  Add19_2 : Sum
  Add20_1 : Sum
  Add2_1 : Sum
  Add3_1 : Sum
  Add4_1 : Sum
  Add5_1 : Sum
  Add6_1 : Sum
  Add7_1 : Sum
  Add8_1 : Sum
  Add8_4 : Sum
  Add9_1 : Sum
  Add9_8 : Sum
  ColConst : Constant  Value=0
  Const10_10 : Constant
  Const10_4 : Constant  Value=0.5
  Const10_5 : Constant
  Const11_6 : Constant  Value=0.5
  Const11_7 : Constant
  Const15_8 : Constant  Value=0.022993
  Const4_4 : Constant  Value=0.5
  Const5_3 : Constant  Value=2
  Const5_6 : Constant  Value=0.5
  Const6_3 : Constant  Value=2.718
  Const6_5 : Constant  Value=2
  Const7_4 : Constant
  Const7_5 : Constant  Value=2.718
  Const8_3 : Constant  Value=2
  Const8_6 : Constant
  Const9_5 : Constant
  Const9_7 : Constant  Value=2
  Div10_11 : Product  Inputs=*/
  Div11_4 : Product  Inputs=*/
  Div12_6 : Product  Inputs=*/
  Div4_3 : Product  Inputs=*/
  Div5_5 : Product  Inputs=*/
  Div9_6 : Product  Inputs=*/
  Mul10_3 : Product
  Mul11_5 : Product
  Mul12_3 : Product
  Mul13_7 : Product
  Mul14_5 : Product
  Mul14_6 : Product
  Mul15_3 : Product
  Mul15_5 : Product
  Mul15_6 : Product
  Mul16_5 : Product
  Mul17_4 : Product
  Mul6_4 : Product
  Mul7_6 : Product
  Pow11_3 : Math  Operator=pow  SaturateOnIntegerOverflow=on
  Pow12_5 : Math  Operator=pow  SaturateOnIntegerOverflow=on
  Pow5_4 : Math  Operator=pow  SaturateOnIntegerOverflow=on
  Pow6_6 : Math  Operator=pow  SaturateOnIntegerOverflow=on
  Pow7_3 : Math  Operator=pow  SaturateOnIntegerOverflow=on
  Pow8_5 : Math  Operator=pow  SaturateOnIntegerOverflow=on
  RowConst : Constant  Value=0
  Sub10_7 : Sum  Inputs=+-
  Sub11_9 : Sum  Inputs=+-
  Sub13_6 : Sum  Inputs=+-
  Sub14_10 : Sum  Inputs=+-
  Row : Outport
  Col : Outport  Port=2
  Value : Outport  Port=3
  wires:
  ColConst/1 -> Col/1
  RowConst/1 -> Row/1
  Add20_1/1 -> Value/1
  Add19_1/1 -> Add20_1/1
  Add18_1/1 -> Add19_1/1
  Add17_1/1 -> Add18_1/1
  Add16_1/1 -> Add17_1/1
  Add15_1/1 -> Add16_1/1
  Add14_1/1 -> Add15_1/1
  Add13_1/1 -> Add14_1/1
  Add12_1/1 -> Add13_1/1
  Add11_1/1 -> Add12_1/1
  Add10_1/1 -> Add11_1/1
  Add9_1/1 -> Add10_1/1
  Add8_1/1 -> Add9_1/1
  Add7_1/1 -> Add8_1/1
  Add6_1/1 -> Add7_1/1
  Add5_1/1 -> Add6_1/1
  Add4_1/1 -> Add5_1/1
  Add3_1/1 -> Add4_1/1
  Add2_1/1 -> Add3_1/1
  [State1] -> Add2_1/1
  [State2] -> Add2_1/2
  [State3] -> Add3_1/2
  [State4] -> Add4_1/2
  [State5] -> Add5_1/2
  [State6] -> Add6_1/2
  [State7] -> Add7_1/2
  [State8] -> Add8_1/2
  [State9] -> Add9_1/2
  [State10] -> Add10_1/2
  [State11] -> Add11_1/2
  [State12] -> Add12_1/2
  [State13] -> Add13_1/2
  [State14] -> Add14_1/2
  [State15] -> Add15_1/2
  [State16] -> Add16_1/2
  [State17] -> Add17_1/2
  [State18] -> Add18_1/2
  [State19] -> Add19_1/2
  Add19_2/1 -> Add20_1/2
  Add18_3/1 -> Add19_2/1
  Add17_3/1 -> Add18_3/1
  Add16_3/1 -> Add17_3/1
  Mul15_3/1 -> Add16_3/1
  [InputCurrent] -> Mul15_3/1
  [ID1_ObjR] -> Mul15_3/2
  Add15_4/1 -> Add16_3/2
  Mul14_5/1 -> Add15_4/1
  [InputCurrent] -> Mul14_5/1
  [ID0_ObjR] -> Mul14_5/2
  Mul14_6/1 -> Add15_4/2
  [InputCurrent] -> Mul14_6/1
  Sub13_6/1 -> Mul14_6/2
  Mul12_3/1 -> Sub13_6/1
  Pow11_3/1 -> Mul12_3/1
  Mul10_3/1 -> Pow11_3/1
  [ID4_ObjCT] -> Mul10_3/1
  [ID4_ObjMP] -> Mul10_3/2
  Const10_4/1 -> Pow11_3/2
  Div11_4/1 -> Mul12_3/2
  Const10_5/1 -> Div11_4/1
  Sub10_7/1 -> Div11_4/2
  Const9_5/1 -> Sub10_7/1
  Div9_6/1 -> Sub10_7/2
  Const8_3/1 -> Div9_6/1
  Add8_4/1 -> Div9_6/2
  Pow7_3/1 -> Add8_4/1
  Const6_3/1 -> Pow7_3/1
  Mul6_4/1 -> Pow7_3/2
  Const5_3/1 -> Mul6_4/1
  Pow5_4/1 -> Mul6_4/2
  Div4_3/1 -> Pow5_4/1
  [ID4_ObjMP] -> Div4_3/1
  [ID4_ObjCT] -> Div4_3/2
  Const4_4/1 -> Pow5_4/2
  Const7_4/1 -> Add8_4/2
  [ID4_ObjCT] -> Sub13_6/2
  Add16_4/1 -> Add17_3/2
  Mul15_5/1 -> Add16_4/1
  [InputCurrent] -> Mul15_5/1
  [ID0_ObjR] -> Mul15_5/2
  Mul15_6/1 -> Add16_4/2
  [InputCurrent] -> Mul15_6/1
  Sub14_10/1 -> Mul15_6/2
  Mul13_7/1 -> Sub14_10/1
  Pow12_5/1 -> Mul13_7/1
  Mul11_5/1 -> Pow12_5/1
  [ID5_ObjCT] -> Mul11_5/1
  [ID5_ObjMP] -> Mul11_5/2
  Const11_6/1 -> Pow12_5/2
  Div12_6/1 -> Mul13_7/2
  Const11_7/1 -> Div12_6/1
  Sub11_9/1 -> Div12_6/2
  Const10_10/1 -> Sub11_9/1
  Div10_11/1 -> Sub11_9/2
  Const9_7/1 -> Div10_11/1
  Add9_8/1 -> Div10_11/2
  Pow8_5/1 -> Add9_8/1
  Const7_5/1 -> Pow8_5/1
  Mul7_6/1 -> Pow8_5/2
  Const6_5/1 -> Mul7_6/1
  Pow6_6/1 -> Mul7_6/2
  Div5_5/1 -> Pow6_6/1
  [ID5_ObjMP] -> Div5_5/1
  [ID5_ObjCT] -> Div5_5/2
  Const5_6/1 -> Pow6_6/2
  Const8_6/1 -> Add9_8/2
  [ID5_ObjCT] -> Sub14_10/2
  Mul17_4/1 -> Add18_3/2
  Mul16_5/1 -> Mul17_4/1
  [InputCurrent] -> Mul16_5/1
  Const15_8/1 -> Mul16_5/2
  [ID6_ObjR] -> Mul17_4/2
  [ID7_ObjV] -> Add19_2/2

== system xEMU_SimulationModel3_rule1/Battery (BAT)_komplex/Subsystem/CellVoltageMatrices/Component1 ==
  Add10_1 : Sum
  Add11_1 : Sum
  Add12_1 : Sum
  Add13_1 : Sum
  Add14_1 : Sum
  Add15_1 : Sum
  Add15_4 : Sum
  Add16_1 : Sum
  Add16_3 : Sum
  Add16_4 : Sum
  Add17_1 : Sum
  Add17_3 : Sum
  Add18_1 : Sum
  Add18_3 : Sum
  Add19_1 : Sum
  Add19_2 : Sum
  Add20_1 : Sum
  Add2_1 : Sum
  Add3_1 : Sum
  Add4_1 : Sum
  Add5_1 : Sum
  Add6_1 : Sum
  Add7_1 : Sum
  Add8_1 : Sum
  Add8_4 : Sum
  Add9_1 : Sum
  Add9_8 : Sum
  ColConst : Constant  Value=0
  Const10_10 : Constant
  Const10_4 : Constant  Value=0.5
  Const10_5 : Constant
  Const11_6 : Constant  Value=0.5
  Const11_7 : Constant
  Const15_8 : Constant  Value=0.022993
  Const4_4 : Constant  Value=0.5
  Const5_3 : Constant  Value=2
  Const5_6 : Constant  Value=0.5
  Const6_3 : Constant  Value=2.718
  Const6_5 : Constant  Value=2
  Const7_4 : Constant
  Const7_5 : Constant  Value=2.718
  Const8_3 : Constant  Value=2
  Const8_6 : Constant
  Const9_5 : Constant
  Const9_7 : Constant  Value=2
  Div10_11 : Product  Inputs=*/
  Div11_4 : Product  Inputs=*/
  Div12_6 : Product  Inputs=*/
  Div4_3 : Product  Inputs=*/
  Div5_5 : Product  Inputs=*/
  Div9_6 : Product  Inputs=*/
  Mul10_3 : Product
  Mul11_5 : Product
  Mul12_3 : Product
  Mul13_7 : Product
  Mul14_5 : Product
  Mul14_6 : Product
  Mul15_3 : Product
  Mul15_5 : Product
  Mul15_6 : Product
  Mul16_5 : Product
  Mul17_4 : Product
  Mul6_4 : Product
  Mul7_6 : Product
  Pow11_3 : Math  Operator=pow  SaturateOnIntegerOverflow=on
  Pow12_5 : Math  Operator=pow  SaturateOnIntegerOverflow=on
  Pow5_4 : Math  Operator=pow  SaturateOnIntegerOverflow=on
  Pow6_6 : Math  Operator=pow  SaturateOnIntegerOverflow=on
  Pow7_3 : Math  Operator=pow  SaturateOnIntegerOverflow=on
  Pow8_5 : Math  Operator=pow  SaturateOnIntegerOverflow=on
  RowConst : Constant  Value=0
  Sub10_7 : Sum  Inputs=+-
  Sub11_9 : Sum  Inputs=+-
  Sub13_6 : Sum  Inputs=+-
  Sub14_10 : Sum  Inputs=+-
  Row : Outport
  Col : Outport  Port=2
  Value : Outport  Port=3
  wires:
  ColConst/1 -> Col/1
  RowConst/1 -> Row/1
  Add20_1/1 -> Value/1
  Add19_1/1 -> Add20_1/1
  Add18_1/1 -> Add19_1/1
  Add17_1/1 -> Add18_1/1
  Add16_1/1 -> Add17_1/1
  Add15_1/1 -> Add16_1/1
  Add14_1/1 -> Add15_1/1
  Add13_1/1 -> Add14_1/1
  Add12_1/1 -> Add13_1/1
  Add11_1/1 -> Add12_1/1
  Add10_1/1 -> Add11_1/1
  Add9_1/1 -> Add10_1/1
  Add8_1/1 -> Add9_1/1
  Add7_1/1 -> Add8_1/1
  Add6_1/1 -> Add7_1/1
  Add5_1/1 -> Add6_1/1
  Add4_1/1 -> Add5_1/1
  Add3_1/1 -> Add4_1/1
  Add2_1/1 -> Add3_1/1
  [State1] -> Add2_1/1
  [State2] -> Add2_1/2
  [State3] -> Add3_1/2
  [State4] -> Add4_1/2
  [State5] -> Add5_1/2
  [State6] -> Add6_1/2
  [State7] -> Add7_1/2
  [State8] -> Add8_1/2
  [State9] -> Add9_1/2
  [State10] -> Add10_1/2
  [State11] -> Add11_1/2
  [State12] -> Add12_1/2
  [State13] -> Add13_1/2
  [State14] -> Add14_1/2
  [State15] -> Add15_1/2
  [State16] -> Add16_1/2
  [State17] -> Add17_1/2
  [State18] -> Add18_1/2
  [State19] -> Add19_1/2
  Add19_2/1 -> Add20_1/2
  Add18_3/1 -> Add19_2/1
  Add17_3/1 -> Add18_3/1
  Add16_3/1 -> Add17_3/1
  Mul15_3/1 -> Add16_3/1
  [InputCurrent] -> Mul15_3/1
  [ID1_ObjR] -> Mul15_3/2
  Add15_4/1 -> Add16_3/2
  Mul14_5/1 -> Add15_4/1
  [InputCurrent] -> Mul14_5/1
  [ID0_ObjR] -> Mul14_5/2
  Mul14_6/1 -> Add15_4/2
  [InputCurrent] -> Mul14_6/1
  Sub13_6/1 -> Mul14_6/2
  Mul12_3/1 -> Sub13_6/1
  Pow11_3/1 -> Mul12_3/1
  Mul10_3/1 -> Pow11_3/1
  [ID4_ObjCT] -> Mul10_3/1
  [ID4_ObjMP] -> Mul10_3/2
  Const10_4/1 -> Pow11_3/2
  Div11_4/1 -> Mul12_3/2
  Const10_5/1 -> Div11_4/1
  Sub10_7/1 -> Div11_4/2
  Const9_5/1 -> Sub10_7/1
  Div9_6/1 -> Sub10_7/2
  Const8_3/1 -> Div9_6/1
  Add8_4/1 -> Div9_6/2
  Pow7_3/1 -> Add8_4/1
  Const6_3/1 -> Pow7_3/1
  Mul6_4/1 -> Pow7_3/2
  Const5_3/1 -> Mul6_4/1
  Pow5_4/1 -> Mul6_4/2
  Div4_3/1 -> Pow5_4/1
  [ID4_ObjMP] -> Div4_3/1
  [ID4_ObjCT] -> Div4_3/2
  Const4_4/1 -> Pow5_4/2
  Const7_4/1 -> Add8_4/2
  [ID4_ObjCT] -> Sub13_6/2
  Add16_4/1 -> Add17_3/2
  Mul15_5/1 -> Add16_4/1
  [InputCurrent] -> Mul15_5/1
  [ID0_ObjR] -> Mul15_5/2
  Mul15_6/1 -> Add16_4/2
  [InputCurrent] -> Mul15_6/1
  Sub14_10/1 -> Mul15_6/2
  Mul13_7/1 -> Sub14_10/1
  Pow12_5/1 -> Mul13_7/1
  Mul11_5/1 -> Pow12_5/1
  [ID5_ObjCT] -> Mul11_5/1
  [ID5_ObjMP] -> Mul11_5/2
  Const11_6/1 -> Pow12_5/2
  Div12_6/1 -> Mul13_7/2
  Const11_7/1 -> Div12_6/1
  Sub11_9/1 -> Div12_6/2
  Const10_10/1 -> Sub11_9/1
  Div10_11/1 -> Sub11_9/2
  Const9_7/1 -> Div10_11/1
  Add9_8/1 -> Div10_11/2
  Pow8_5/1 -> Add9_8/1
  Const7_5/1 -> Pow8_5/1
  Mul7_6/1 -> Pow8_5/2
  Const6_5/1 -> Mul7_6/1
  Pow6_6/1 -> Mul7_6/2
  Div5_5/1 -> Pow6_6/1
  [ID5_ObjMP] -> Div5_5/1
  [ID5_ObjCT] -> Div5_5/2
  Const5_6/1 -> Pow6_6/2
  Const8_6/1 -> Add9_8/2
  [ID5_ObjCT] -> Sub14_10/2
  Mul17_4/1 -> Add18_3/2
  Mul16_5/1 -> Mul17_4/1
  [InputCurrent] -> Mul16_5/1
  Const15_8/1 -> Mul16_5/2
  [ID6_ObjR] -> Mul17_4/2
  [ID7_ObjV] -> Add19_2/2
